simulink model "scheme1"  (R2024a)
settings: Solver=VariableStepAuto  StartTime=0.0  StopTime=10.0  RelTol=1e-8
undefined symbols (not defined in the file or in its folder): A, B, Bf, Cz, Gamma, K1, K2, wfen, x0
settings Model: Creator=alexivanov  LastModifiedBy=alexivanov

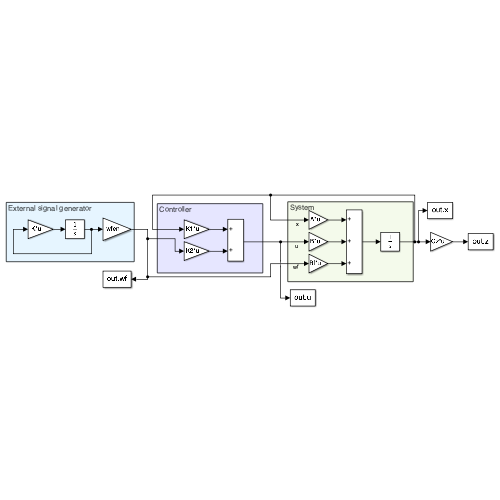
[thumbnail: Simulink's stored preview of the top-level diagram]
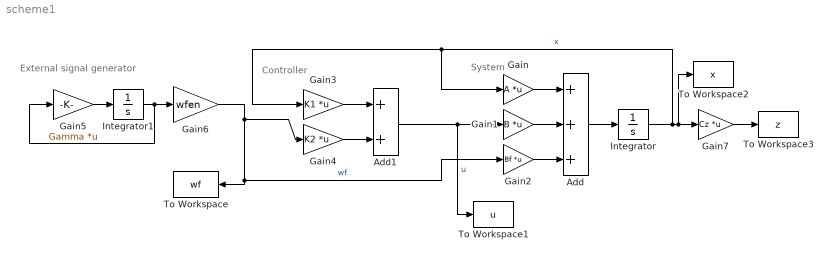
== system scheme1 ==
  note: System
  note: External signal generator
  note: Controller
  Add : Sum  Inputs=+++
  Add1 : Sum
  Gain : Gain  Gain=A  Multiplication=Matrix(K*u)
  Gain1 : Gain  Gain=B  Multiplication=Matrix(K*u)
  Gain2 : Gain  Gain=Bf  Multiplication=Matrix(K*u)
  Gain3 : Gain  Gain=K1  Multiplication=Matrix(K*u)
  Gain4 : Gain  Gain=K2  Multiplication=Matrix(K*u)
  Gain5 : Gain  Gain=Gamma  Multiplication=Matrix(K*u)
  Gain6 : Gain  Gain=wfen
  Gain7 : Gain  Gain=Cz  Multiplication=Matrix(K*u)
  Integrator : Integrator  InitialCondition=x0
  Integrator1 : Integrator  InitialCondition=[1; 1; 1; 1]
  To Workspace : ToWorkspace  VariableName=wf  SampleTime=-1
  To Workspace1 : ToWorkspace  VariableName=u  SampleTime=-1
  To Workspace2 : ToWorkspace  VariableName=x  SampleTime=-1
  To Workspace3 : ToWorkspace  VariableName=z  SampleTime=-1
  wires:
  Add/1 -> Integrator/1
  Gain/1 -> Add/1
  Gain1/1 -> Add/2
  Gain2/1 -> Add/3
  Integrator/1 -> Gain7/1, To Workspace2/1, Gain3/1, Gain/1  "x"
  Gain3/1 -> Add1/1
  Gain4/1 -> Add1/2
  Add1/1 -> To Workspace1/1, Gain1/1  "u"
  Gain5/1 -> Integrator1/1
  Integrator1/1 -> Gain5/1, Gain6/1
  Gain6/1 -> Gain4/1, To Workspace/1, Gain2/1  "wf"
  Gain7/1 -> To Workspace3/1
